simulink model "SignalBuilder"  (R2018a)
settings: Solver=ode23tb  StartTime=0.0  StopTime=0.15  MaxStep=10e-6  RelTol=1e-3
undefined symbols (not defined in the file): sigbuilder_block
settings Model: Creator=ivank  LastModifiedBy=ivank
settings SolverCC: InitialStep=10e-8

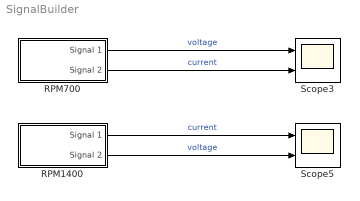
== system SignalBuilder ==
  RPM1400 : Subsystem  Tag=STV Subsys  LoadFcn=sigbuilder_block('load');  StartFcn=sigbuilder_block('start');  StopFcn=sigbuilder_block('stop');  ClipboardFcn=sigbuilder_block('clipboard');  mask(Sigbuilder block){tuvar=[0:10]}
      mask help: Simulink:masks:SigbuilderBlock_MD
      mask init:
      | if ~strcmp(get_param(bdroot(gcbh),'SimulationStatus'),'stopped') tuvar = sigbuilder_block('maskInit'); end
      settings: CopyFcn=sigbuilder_block('copy');  DeleteFcn=sigbuilder_block('delete');  ModelCloseFcn=sigbuilder_block('modelClose');  PreSaveFcn=sigbuilder_block('preSave');  PauseFcn=sigbuilder_block('pause');  ContinueFcn=sigbuilder_block('continue');  NameChangeFcn=sigbuilder_block('namechange');  OpenFcn=sigbuilder_block('open',[352.2 1.2 475.2 479.4 ]);  CloseFcn=sigbuilder_block('close');
      mask Display: plot(0, 0, 100, 100,[2, 2, 32, 32, 2], [68, 8, 8, 68, 68],[32, 2], [38, 38], [32, 19, 2],[53, 60, 44], [32, 17, 17, 2],[16, 16, 31, 31]);txt = getActiveGroup(gcbh);text(2, 100, txt,'verticalAlignment', 'top');
  RPM700 : Subsystem  Tag=STV Subsys  LoadFcn=sigbuilder_block('load');  StartFcn=sigbuilder_block('start');  StopFcn=sigbuilder_block('stop');  ClipboardFcn=sigbuilder_block('clipboard');  mask(Sigbuilder block){tuvar=[0:10]}
      mask help: Simulink:masks:SigbuilderBlock_MD
      mask init:
      | if ~strcmp(get_param(bdroot(gcbh),'SimulationStatus'),'stopped') tuvar = sigbuilder_block('maskInit'); end
      settings: CopyFcn=sigbuilder_block('copy');  DeleteFcn=sigbuilder_block('delete');  ModelCloseFcn=sigbuilder_block('modelClose');  PreSaveFcn=sigbuilder_block('preSave');  PauseFcn=sigbuilder_block('pause');  ContinueFcn=sigbuilder_block('continue');  NameChangeFcn=sigbuilder_block('namechange');  OpenFcn=sigbuilder_block('open',[507 100.8 550.8 360 ]);  CloseFcn=sigbuilder_block('close');
      mask Display: plot(0, 0, 100, 100,[2, 2, 32, 32, 2], [68, 8, 8, 68, 68],[32, 2], [38, 38], [32, 19, 2],[53, 60, 44], [32, 17, 17, 2],[16, 16, 31, 31]);txt = getActiveGroup(gcbh);text(2, 100, txt,'verticalAlignment', 'top');
  Scope3 : Scope  NumInputPorts=2
  Scope5 : Scope  NumInputPorts=2
  wires:
  RPM1400/2(Signal 2) -> Scope5/2  "voltage"
  RPM1400/1(Signal 1) -> Scope5/1  "current"
  RPM700/1(Signal 1) -> Scope3/1  "voltage"
  RPM700/2(Signal 2) -> Scope3/2  "current"

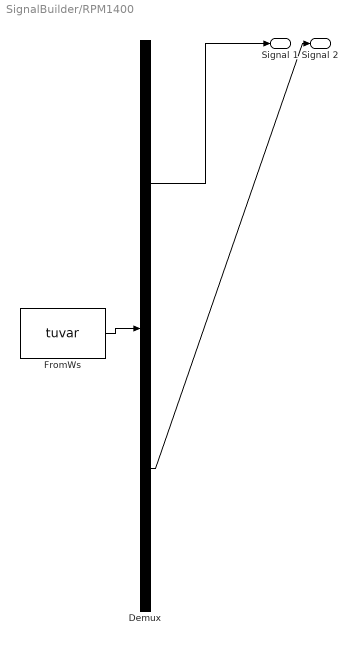
== system SignalBuilder/RPM1400 ==
  Demux : Demux  Tag=STV Demux  Outputs=2
  FromWs : FromWorkspace  Tag=STV FromWs  VariableName=tuvar  SampleTime=0
      SigBuilderData=|
      | common.afterFinalStr = 'Extrapolate'
      | common.sampleTime = 0
      | dataSet.timeRange = [0 0.0999992]
      | dataSet.name = 'Group 1'
      | sbobj.Groups.Name = 'Group 1'
      | sbobj.Groups.Signals(1).Name = 'Signal 1'
      | sbobj.Groups.Signals(1).XData = [0 8.00000000002e-07 1.6e-06 2.4e-06 3.2e-06 4e-06 4.80000000001e-06 5.6e-06 6.4e-06 7.20000000001e-06 8e-06 8.8e-06 ... (125000 elements, 1x125000)]
      | sbobj.Groups.Signals(1).YData = [-2.7 -2.5 -2.5 -2.5 -2.7 -2.5 -2.5 -2.5 -2.7 -2.7 -2.7 -2.5 ... (125000 elements, 1x125000)]
      | sbobj.Groups.Signals(2).Name = 'Signal 2'
      | sbobj.Groups.Signals(2).XData = [0 8.00000000002e-07 1.6e-06 2.4e-06 3.2e-06 4e-06 4.80000000001e-06 5.6e-06 6.4e-06 7.20000000001e-06 8e-06 8.8e-06 ... (125000 elements, 1x125000)]
      | sbobj.Groups.Signals(2).YData = [20 20 60 -20 20 -20 20 20 20 20 20 20 ... (125000 elements, 1x125000)]
      | sbobj.Groups.TimeRange = [0 0.0999992]
  Signal 1 : Outport  Tag=STV Outport
  Signal 2 : Outport  Tag=STV Outport  Port=2
  wires:
  Demux/1 -> Signal 1/1
  FromWs/1 -> Demux/1
  Demux/2 -> Signal 2/1

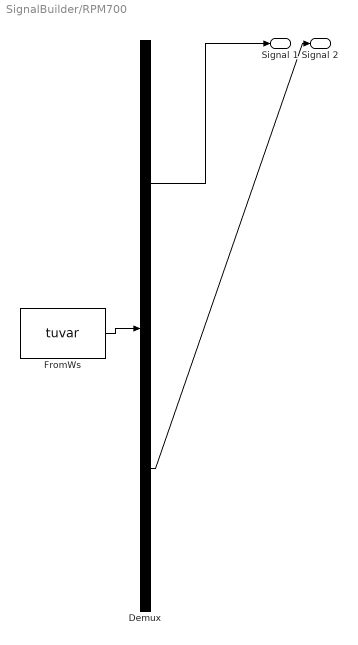
== system SignalBuilder/RPM700 ==
  Demux : Demux  Tag=STV Demux  Outputs=2
  FromWs : FromWorkspace  Tag=STV FromWs  VariableName=tuvar  SampleTime=0
      SigBuilderData=|
      | common.afterFinalStr = 'Extrapolate'
      | common.sampleTime = 0
      | dataSet.timeRange = [0 0.15]
      | dataSet.name = 'Group 1'
      | sbobj.Groups.Name = 'Group 1'
      | sbobj.Groups.Signals(1).Name = 'Signal 1'
      | sbobj.Groups.Signals(1).XData = [0 8.00000000002e-07 1.6e-06 2.4e-06 3.2e-06 4e-06 4.80000000001e-06 5.6e-06 6.4e-06 7.20000000001e-06 8e-06 8.8e-06 ... (125000 elements, 1x125000)]
      | sbobj.Groups.Signals(1).YData = [20 20 20 20 20 20 20 20 20 20 20 20 ... (125000 elements, 1x125000)]
      | sbobj.Groups.Signals(2).Name = 'Signal 2'
      | sbobj.Groups.Signals(2).XData = [0 8.00000000002e-07 1.6e-06 2.4e-06 3.2e-06 4e-06 4.80000000001e-06 5.6e-06 6.4e-06 7.20000000001e-06 8e-06 8.8e-06 ... (125000 elements, 1x125000)]
      | sbobj.Groups.Signals(2).YData = [-1.7 -2.1 -1.9 -1.9 -1.9 -1.9 -1.9 -1.9 -2.1 -1.9 -2.1 -2.1 ... (125000 elements, 1x125000)]
      | sbobj.Groups.TimeRange = [0 0.15]
  Signal 1 : Outport  Tag=STV Outport
  Signal 2 : Outport  Tag=STV Outport  Port=2
  wires:
  Demux/1 -> Signal 1/1
  FromWs/1 -> Demux/1
  Demux/2 -> Signal 2/1
